simulink library "Electrical_to_Mechanical_gen"  (R2016a)
settings: Solver=ode45  StartTime=0.0  StopTime=10.0  RelTol=1e-3
undefined symbols (not defined in the file): API1dcac_efficiency, API2dcac_efficiency, API3dcac_efficiency, APIdcac_efficiency, aux_power_state, auxEmot_inertia, auxEmot_nTab_3rdD, auxEmot_power, auxEmot_pwrAC, auxEmot_Tau, auxEmot_trqTab_2ndD, auxEmot_vltTab_1stD, AWR_InvStError, DiscIntNeverNeededParam, drvEmot_emot_Cth_rotor, drvEmot_emot_Cth_stator, drvEmot_emot_dtrqEmotNeg, drvEmot_emot_dtrqEmotPtv, drvEmot_emot_inv_pwrLoss, drvEmot_emot_mot_pwrLoss, drvEmot_emot_Rth_rotor_oil, drvEmot_emot_Rth_stator_oil, drvEmot_emot_Rth_stator_rotor, drvEmot_emot_Trotor_init, drvEmot_emot_trqMaxRow, drvEmot_emot_trqMinRow, drvEmot_emot_Tstator_init, drvEmot_inv_Cth_cooling_plate, drvEmot_inv_Cth_diode, drvEmot_inv_Cth_IGBT, drvEmot_inv_n_IGBT_per_Switch, drvEmot_inv_Rth_cooling_plate_coolant, drvEmot_inv_Rth_PS_cooling_plate, drvEmot_inv_Tplate_init, drvEmot_inv_Tpowerstack_init, drvEmot_RefTqeMOT, emot_AcCmprFront_inertia, emot_AcCmprFront_nTab_3rdD, emot_AcCmprFront_pwrAC, emot_AcCmprFront_Tau, emot_AcCmprFront_trqTab_2ndD, emot_AcCmprFront_vltTab_1stD, emot_AcCmprRear_inertia, emot_AcCmprRear_nTab_3rdD, emot_AcCmprRear_pwrAC, emot_AcCmprRear_Tau, emot_AcCmprRear_trqTab_2ndD, emot_AcCmprRear_vltTab_1stD, emot_AirCmpr_inertia, emot_AirCmpr_nTab_3rdD, emot_AirCmpr_pwrAC, emot_AirCmpr_Tau, emot_AirCmpr_trqTab_2ndD, emot_AirCmpr_vltTab_1stD, emot_aircomp_power, FirstDrivenAxle_FirstDrivenAxleNoOfEmot, SecondDrivenAxle_SecondDrivenAxleNoOfEmot
libraries: Electrical_to_Mechanical_gen x4, simulink x4
(part 1 of 2)
settings Model: Creator=krishs1  LastModifiedBy=krishs1
settings DataIOCC: LimitDataPoints=on
settings DebuggingCC: AllowSymbolicDim=off

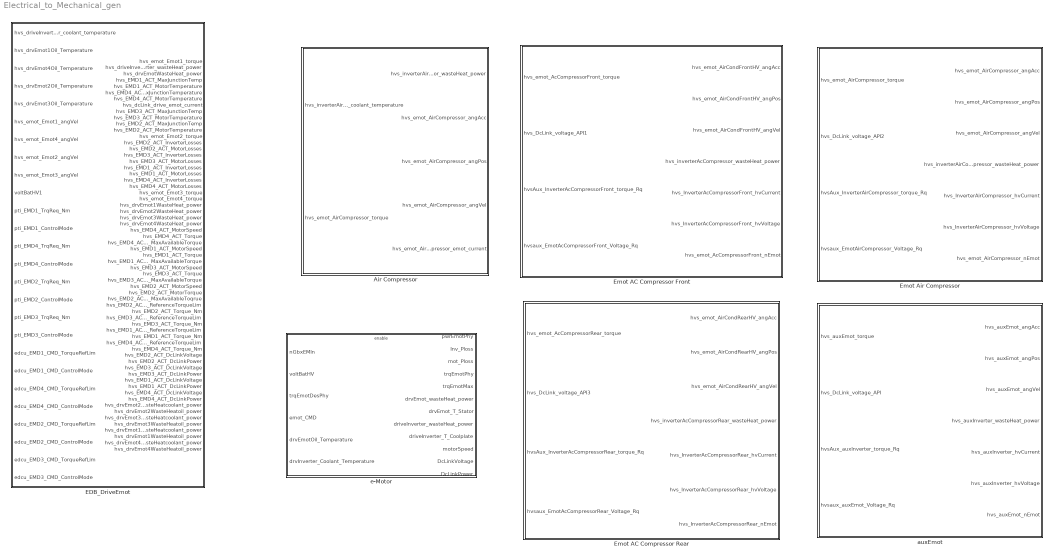
== system Electrical_to_Mechanical_gen ==
  Air Compressor : Subsystem
  EDB_DriveEmot : Subsystem
  Emot AC Compressor Front : Subsystem
  Emot AC Compressor Rear : Subsystem
  Emot Air Compressor : Subsystem
  auxEmot : Subsystem  mask{auxEmot_nTab_3rdD=auxEmot_nTab_3rdD, auxEmot_trqTab_2ndD=auxEmot_trqTab_2ndD, auxEmot_vltTab_1stD=auxEmot_vltTab_1stD, auxEmot_pwrAC=auxEmot_pwrAC, APIefficiency=1/APIdcac_efficiency, auxEmot_inertia=auxEmot_inertia, auxEmot_Tau=auxEmot_Tau, AWR_InvStError=AWR_InvStError, auxEmot_power=auxEmot_power, aux_power_state=aux_power_state}
      mask prompts: auxEmot_nTab_3rdD "Motor speed"; auxEmot_trqTab_2ndD "Motor torque"; auxEmot_vltTab_1stD "Motor voltage"; auxEmot_pwrAC "Motor power map"; APIefficiency "API efficiency"; auxEmot_inertia "Motor inertia"; AWR_InvStError "Inverter state error"; auxEmot_power "Motor average power"; aux_power_state "Switch real or constant load"
      mask TypeOptions auxEmot_nTab_3rdD: motor mode/BreakpointsForDimension1
      mask TypeOptions auxEmot_trqTab_2ndD: motor mode/BreakpointsForDimension2
      mask TypeOptions auxEmot_vltTab_1stD: motor mode/BreakpointsForDimension3
      mask TypeOptions auxEmot_pwrAC: motor mode/Table
      mask TypeOptions APIefficiency: efficiency/Gain
      mask TypeOptions auxEmot_inertia: auxEmot_inertia/Value
      mask TypeOptions AWR_InvStError: AWR_InvStError/const
      mask TypeOptions auxEmot_power: lvs_Aircomp_power/Value
      mask TypeOptions aux_power_state: switch_Real_or_Constant_Load/Value
  e-Motor : Subsystem  mask(MapModule){}

== system Electrical_to_Mechanical_gen/Air Compressor ==
  hvs_inverterAirCompressor_coolant_temperature : Inport
  hvs_emot_AirCompressor_torque : Inport  Port=2
  Constant{,1..4} (5 alike) : Constant  Value=0
  Terminator : Terminator
  Terminator1 : Terminator
  "hvs_inverterAirCompressor_wasteHeat_power " : Outport
  hvs_emot_AirCompressor_angAcc : Outport  Port=2
  hvs_emot_AirCompressor_angPos : Outport  Port=3
  hvs_emot_AirCompressor_angVel : Outport  Port=4
  hvs_emot_AirCompressor_emot_current : Outport  Port=5
  wires:
  Constant/1 -> "hvs_inverterAirCompressor_wasteHeat_power "/1
  Constant1/1 -> hvs_emot_AirCompressor_angAcc/1
  Constant2/1 -> hvs_emot_AirCompressor_angPos/1
  Constant3/1 -> hvs_emot_AirCompressor_angVel/1
  Constant4/1 -> hvs_emot_AirCompressor_emot_current/1
  hvs_inverterAirCompressor_coolant_temperature/1 -> Terminator/1
  hvs_emot_AirCompressor_torque/1 -> Terminator1/1

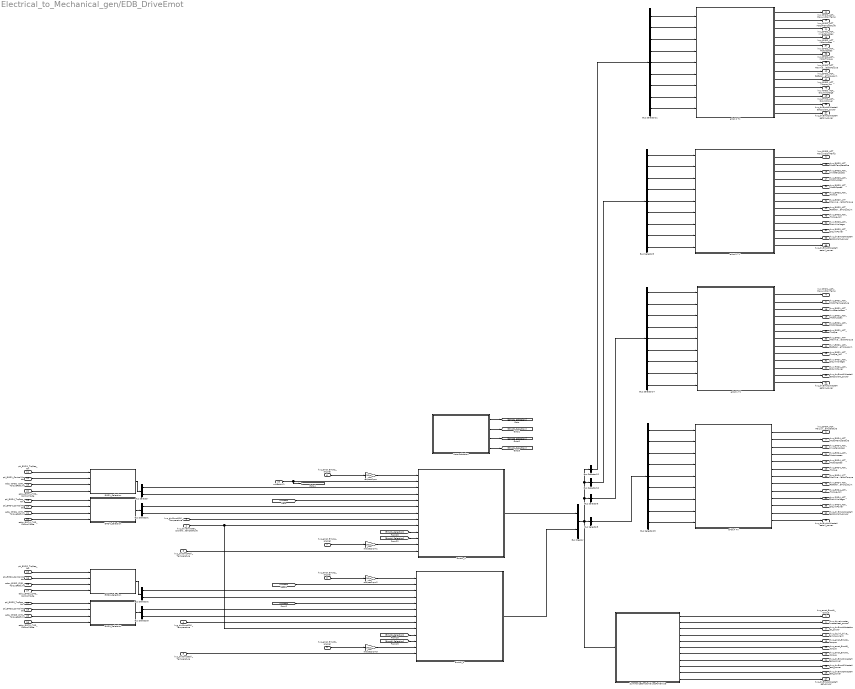
== system Electrical_to_Mechanical_gen/EDB_DriveEmot ==
  hvs_driveInverter_coolant_temperature : Inport
  hvs_drvEmot1Oil_Temperature : Inport  Port=2
  hvs_drvEmot4Oil_Temperature : Inport  Port=3
  hvs_drvEmot2Oil_Temperature : Inport  Port=4
  hvs_drvEmot3Oil_Temperature : Inport  Port=5
  hvs_emot_Emot1_angVel : Inport  Port=6
  hvs_emot_Emot4_angVel : Inport  Port=7
  hvs_emot_Emot2_angVel : Inport  Port=8
  hvs_emot_Emot3_angVel : Inport  Port=9
  voltBatHV1 : Inport  Port=10
  pti_EMD1_TrqReq_Nm : Inport  Port=11
  pti_EMD1_ControlMode : Inport  Port=12
  pti_EMD4_TrqReq_Nm : Inport  Port=13
  pti_EMD4_ControlMode : Inport  Port=14
  pti_EMD2_TrqReq_Nm : Inport  Port=15
  pti_EMD2_ControlMode : Inport  Port=16
  pti_EMD3_TrqReq_Nm : Inport  Port=17
  pti_EMD3_ControlMode : Inport  Port=18
  edcu_EMD1_CMD_TorqueRefLim : Inport  Port=19
  edcu_EMD1_CMD_ControlMode : Inport  Port=20
  edcu_EMD4_CMD_TorqueRefLim : Inport  Port=21
  edcu_EMD4_CMD_ControlMode : Inport  Port=22
  edcu_EMD2_CMD_TorqueRefLim : Inport  Port=23
  edcu_EMD2_CMD_ControlMode : Inport  Port=24
  edcu_EMD3_CMD_TorqueRefLim : Inport  Port=25
  edcu_EMD3_CMD_ControlMode : Inport  Port=26
  Bus Selector : BusSelector  OutputSignals=EMD1_TrqReq_Nm,EMD1_ControlMode
  Bus Selector1 : BusSelector  OutputSignals=EMD4_TrqReq_Nm,EMD4_ControlMode
  Bus Selector{9,11,14..15} (4 alike) : BusSelector  OutputSignals=driveInverter_T_plate,drvEmot_T_Stator,Inv_Ploss,mot_Ploss,motorSpeed,trqEmotPhy,trqEmotMax,DcLinkVoltage,DcLinkPower
  Bus Selector2 : BusSelector  OutputSignals=EMD2_TrqReq_Nm,EMD2_ControlMode
  Bus Selector3 : BusSelector  OutputSignals=EMD2_TrqReq_Nm,EMD2_ControlMode
  Bus Creator : BusCreator  Inputs=2
  Bus Selector10 : BusSelector  OutputSignals=emot2_3B.emot3B.driveInverter_T_plate,emot2_3B.emot3B.drvEmot_T_Stator,emot2_3B.emot3B.Inv_Ploss,emot2_3B.emot3B.mot_Ploss,emot2_3B.emot3B.motorSpeed,emot2_3B.emot3B.trqEmotPhy,emot2_3B.emot3B.trqEmotMax,emot2_3B.emot3B.DcLinkVoltage,emot2_3B.emot3B.DcLinkPower  OutputAsBus=on
  Bus Selector12 : BusSelector  OutputSignals=emot2_3B.emot2B.driveInverter_T_plate,emot2_3B.emot2B.drvEmot_T_Stator,emot2_3B.emot2B.Inv_Ploss,emot2_3B.emot2B.mot_Ploss,emot2_3B.emot2B.motorSpeed,emot2_3B.emot2B.trqEmotPhy,emot2_3B.emot2B.trqEmotMax,emot2_3B.emot2B.DcLinkVoltage,emot2_3B.emot2B.DcLinkPower  OutputAsBus=on
  Bus Selector5 : BusSelector  OutputSignals=emot1_4B.emot4B.motorSpeed,emot1_4B.emot4B.trqEmotPhy,emot1_4B.emot4B.trqEmotMax,emot1_4B.emot4B.driveInverter_T_plate,emot1_4B.emot4B.drvEmot_T_Stator,emot1_4B.emot4B.Inv_Ploss,emot1_4B.emot4B.mot_Ploss,emot1_4B.emot4B.DcLinkVoltage,emot1_4B.emot4B.DcLinkPower  OutputAsBus=on
  Bus Selector6 : BusSelector  OutputSignals=emot1_4B.emot1B.driveInverter_T_plate,emot1_4B.emot1B.drvEmot_T_Stator,emot1_4B.emot1B.Inv_Ploss,emot1_4B.emot1B.mot_Ploss,emot1_4B.emot1B.motorSpeed,emot1_4B.emot1B.trqEmotPhy,emot1_4B.emot1B.trqEmotMax,emot1_4B.emot1B.DcLinkVoltage,emot1_4B.emot1B.DcLinkPower  OutputAsBus=on
  EMD1_Selection : Subsystem
  EMD2_Selection : Subsystem
  EMD3_Selection : Subsystem
  EMD4_Selection : Subsystem
  Emot1_4 : Subsystem
  Emot2_3 : Subsystem
  MotorSelection : Subsystem
  SummarizeEmotorValuesForVehicle : Subsystem  TreatAsAtomicUnit=on
  eMot 1 TX : Subsystem
  eMot 2 TX : Subsystem
  eMot 3 TX : Subsystem
  eMot 4 TX : Subsystem
  rad/sec2rpm{,1..3} (4 alike) : Gain  Gain=30/pi
  hvs_emot_Emot1_torque : Outport
  hvs_driveInverter_wasteHeat_power : Outport  Port=2
  hvs_drvEmotWasteHeat_power : Outport  Port=3
  hvs_EMD1_ACT_MaxJunctionTemp : Outport  Port=4
  hvs_EMD1_ACT_MotorTemperature : Outport  Port=5
  hvs_EMD4_ACT_MaxJunctionTemperature : Outport  Port=6
  hvs_EMD4_ACT_MotorTemperature : Outport  Port=7
  hvs_dcLink_drive_emot_current : Outport  Port=8
  hvs_EMD3_ACT_MaxJunctionTemp : Outport  Port=9
  hvs_EMD3_ACT_MotorTemperature : Outport  Port=10
  hvs_EMD2_ACT_MaxJunctionTemp : Outport  Port=11
  hvs_EMD2_ACT_MotorTemperature : Outport  Port=12
  hvs_emot_Emot2_torque : Outport  Port=13
  hvs_EMD2_ACT_InverterLosses : Outport  Port=14
  hvs_EMD2_ACT_MotorLosses : Outport  Port=15
  hvs_EMD3_ACT_InverterLosses : Outport  Port=16
  hvs_EMD3_ACT_MotorLosses : Outport  Port=17
  hvs_EMD1_ACT_InverterLosses : Outport  Port=18
  hvs_EMD1_ACT_MotorLosses : Outport  Port=19
  hvs_EMD4_ACT_InverterLosses : Outport  Port=20
  hvs_EMD4_ACT_MotorLosses : Outport  Port=21
  hvs_emot_Emot3_torque : Outport  Port=22
  hvs_emot_Emot4_torque : Outport  Port=23
  hvs_drvEmot1WasteHeat_power : Outport  Port=24
  hvs_drvEmot2WasteHeat_power : Outport  Port=25
  hvs_drvEmot3WasteHeat_power : Outport  Port=26
  hvs_drvEmot4WasteHeat_power : Outport  Port=27
  hvs_EMD4_ACT_MotorSpeed : Outport  Port=28
  hvs_EMD4_ACT_Torque : Outport  Port=29
  hvs_EMD4_ACT_MaxAvailableTorque : Outport  Port=30
  hvs_EMD1_ACT_MotorSpeed : Outport  Port=31
  hvs_EMD1_ACT_Torque : Outport  Port=32
  hvs_EMD1_ACT_MaxAvailableTorque : Outport  Port=33
  hvs_EMD3_ACT_MotorSpeed : Outport  Port=34
  hvs_EMD3_ACT_Torque : Outport  Port=35
  hvs_EMD3_ACT_MaxAvailableTorque : Outport  Port=36
  hvs_EMD2_ACT_MotorSpeed : Outport  Port=37
  hvs_EMD2_ACT_MotorTorque : Outport  Port=38
  hvs_EMD2_ACT_MaxAvailableToqrue : Outport  Port=39
  hvs_EMD2_ACT_ReferenceTorqueLim : Outport  Port=40
  hvs_EMD2_ACT_Torque_Nm : Outport  Port=41
  hvs_EMD3_ACT_ReferenceTorqueLim : Outport  Port=42
  hvs_EMD3_ACT_Torque_Nm : Outport  Port=43
  hvs_EMD1_ACT_ReferenceTorqueLim : Outport  Port=44
  hvs_EMD1_ACT_Torque_Nm : Outport  Port=45
  hvs_EMD4_ACT_ReferenceTorqueLim : Outport  Port=46
  hvs_EMD4_ACT_Torque_Nm : Outport  Port=47
  hvs_EMD2_ACT_DcLinkVoltage : Outport  Port=48
  hvs_EMD2_ACT_DcLinkPower : Outport  Port=49
  hvs_EMD3_ACT_DcLinkVoltage : Outport  Port=50
  hvs_EMD3_ACT_DcLinkPower : Outport  Port=51
  hvs_EMD1_ACT_DcLinkVoltage : Outport  Port=52
  hvs_EMD1_ACT_DcLinkPower : Outport  Port=53
  hvs_EMD4_ACT_DcLinkVoltage : Outport  Port=54
  hvs_EMD4_ACT_DcLinkPower : Outport  Port=55
  hvs_drvEmot2WasteHeatcoolant_power : Outport  Port=56
  hvs_drvEmot2WasteHeatoil_power : Outport  Port=57
  hvs_drvEmot3WasteHeatcoolant_power : Outport  Port=58
  hvs_drvEmot3WasteHeatoil_power : Outport  Port=59
  hvs_drvEmot1WasteHeatcoolant_power : Outport  Port=60
  hvs_drvEmot1WasteHeatoil_power : Outport  Port=61
  hvs_drvEmot4WasteHeatcoolant_power : Outport  Port=62
  hvs_drvEmot4WasteHeatoil_power : Outport  Port=63
  wires:
  eMot 4 TX/11(hvs_EMD4_ACT_DcLinkPower) -> hvs_EMD4_ACT_DcLinkPower/1
  eMot 4 TX/10(hvs_EMD4_ACT_DcLinkVoltage) -> hvs_EMD4_ACT_DcLinkVoltage/1
  Bus Selector15/9 -> eMot 4 TX/9(IN_EMD4_ACT_DcLinkPower)  "<DcLinkPower>"
  Bus Selector15/8 -> eMot 4 TX/8(IN_EMD4_ACT_DcLinkVoltage)  "<DcLinkVoltage>"
  eMot 1 TX/11(hvs_EMD1_ACT_DcLinkPower) -> hvs_EMD1_ACT_DcLinkPower/1
  eMot 1 TX/10(hvs_EMD1_ACT_DcLinkVoltage) -> hvs_EMD1_ACT_DcLinkVoltage/1
  Bus Selector14/9 -> eMot 1 TX/9(IN_EMD1_ACT_DcLinkPower)  "<DcLinkPower>"
  Bus Selector14/8 -> eMot 1 TX/8(IN_EMD1_ACT_DcLinkVoltage)  "<DcLinkVoltage>"
  eMot 3 TX/11(hvs_EMD3_ACT_DcLinkPower) -> hvs_EMD3_ACT_DcLinkPower/1
  eMot 3 TX/10(hvs_EMD3_ACT_DcLinkVoltage) -> hvs_EMD3_ACT_DcLinkVoltage/1
  Bus Selector9/8 -> eMot 3 TX/8(IN_EMD3_ACT_DcLinkVoltage)  "<DcLinkVoltage>"
  Bus Selector9/9 -> eMot 3 TX/9(IN_EMD3_ACT_DcLinkPower)  "<DcLinkPower>"
  eMot 2 TX/11(hvs_EMD2_ACT_DcLinkPower) -> hvs_EMD2_ACT_DcLinkPower/1
  eMot 2 TX/10(hvs_EMD2_ACT_DcLinkVoltage) -> hvs_EMD2_ACT_DcLinkVoltage/1
  Bus Selector11/9 -> eMot 2 TX/9(IN_EMD2_ACT_DcLinkPower)  "<DcLinkPower>"
  Bus Selector11/8 -> eMot 2 TX/8(IN_EMD2_ACT_DcLinkVoltage)  "<DcLinkVoltage>"
  Bus Selector2/2 -> Emot2_3/4(emot_CMD2)  "<EMD2_ControlMode>"
  Bus Selector2/1 -> Emot2_3/3(trqEmotDesPhy2)  "<EMD2_TrqReq_Nm>"
  Bus Selector3/1 -> Emot2_3/6(trqEmotDesPhy3)  "<EMD2_TrqReq_Nm>"
  Bus Selector3/2 -> Emot2_3/7(emot_CMD3)  "<EMD2_ControlMode>"
  pti_EMD3_ControlMode/1 -> EMD3_Selection/2(pti_EMD2_ControlMode)
  pti_EMD3_TrqReq_Nm/1 -> EMD3_Selection/1(pti_EMD2_TrqReq_Nm)
  EMD3_Selection/1(Signal) -> Bus Selector3/1
  edcu_EMD3_CMD_ControlMode/1 -> EMD3_Selection/4(edcu_EMD2_CMD_ControlMode)
  edcu_EMD3_CMD_TorqueRefLim/1 -> EMD3_Selection/3(edcu_EMD2_CMD_TorqueRefLim)
  EMD2_Selection/1(Signal) -> Bus Selector2/1
  edcu_EMD2_CMD_ControlMode/1 -> EMD2_Selection/4(edcu_EMD2_CMD_ControlMode)
  edcu_EMD2_CMD_TorqueRefLim/1 -> EMD2_Selection/3(edcu_EMD2_CMD_TorqueRefLim)
  pti_EMD2_ControlMode/1 -> EMD2_Selection/2(pti_EMD2_ControlMode)
  pti_EMD2_TrqReq_Nm/1 -> EMD2_Selection/1(pti_EMD2_TrqReq_Nm)
  Bus Selector1/2 -> Emot1_4/7(emot_CMD4)  "<EMD4_ControlMode>"
  Bus Selector1/1 -> Emot1_4/6(trqEmotDesPhy4)  "<EMD4_TrqReq_Nm>"
  EMD4_Selection/1(Signal) -> Bus Selector1/1
  edcu_EMD4_CMD_ControlMode/1 -> EMD4_Selection/4(edcu_EMD4_CMD_ControlMode)
  edcu_EMD4_CMD_TorqueRefLim/1 -> EMD4_Selection/3(edcu_EMD4_CMD_TorqueRefLim)
  Bus Selector/2 -> Emot1_4/4(emot_CMD1)  "<EMD1_ControlMode>"
  Bus Selector/1 -> Emot1_4/3(trqEmotDesPhy1)  "<EMD1_TrqReq_Nm>"
  EMD1_Selection/1(Signal) -> Bus Selector/1
  edcu_EMD1_CMD_ControlMode/1 -> EMD1_Selection/4(edcu_EMD1_CMD_ControlMode)
  edcu_EMD1_CMD_TorqueRefLim/1 -> EMD1_Selection/3(edcu_EMD1_CMD_TorqueRefLim)
  pti_EMD1_ControlMode/1 -> EMD1_Selection/2(pti_EMD1_ControlMode)
  pti_EMD1_TrqReq_Nm/1 -> EMD1_Selection/1(pti_EMD1_TrqReq_Nm)
  eMot 4 TX/9(hvs_EMD4_ACT_Torque_Nm) -> hvs_EMD4_ACT_Torque_Nm/1
  eMot 4 TX/8(hvs_EMD4_ACT_ReferenceTorqueLim) -> hvs_EMD4_ACT_ReferenceTorqueLim/1
  eMot 1 TX/9(hvs_EMD1_ACT_Torque_Nm) -> hvs_EMD1_ACT_Torque_Nm/1
  eMot 1 TX/8(hvs_EMD1_ACT_ReferenceTorqueLim) -> hvs_EMD1_ACT_ReferenceTorqueLim/1
  eMot 3 TX/9(hvs_EMD3_ACT_Torque_Nm) -> hvs_EMD3_ACT_Torque_Nm/1
  eMot 3 TX/8(hvs_EMD3_ACT_ReferenceTorqueLim) -> hvs_EMD3_ACT_ReferenceTorqueLim/1
  eMot 2 TX/8(hvs_EMD2_ACT_ReferenceTorqueLim) -> hvs_EMD2_ACT_ReferenceTorqueLim/1
  eMot 2 TX/9(hvs_EMD2_ACT_Torque_Nm) -> hvs_EMD2_ACT_Torque_Nm/1
  rad/sec2rpm3/1 -> Emot2_3/12(hvs_emot_Emot3_angVel)
  rad/sec2rpm2/1 -> Emot2_3/1(hvs_emot_Emot2_angVel)
  rad/sec2rpm1/1 -> Emot1_4/12(hvs_emot_Emot4_angVel)
  rad/sec2rpm/1 -> Emot1_4/1(hvs_emot_Emot1_angVel)
  [voltBat] -> Emot2_3/5(voltBatHV3)
  [voltBat] -> Emot2_3/2(voltBatHV2)
  pti_EMD4_ControlMode/1 -> EMD4_Selection/2(pti_EMD4_ControlMode)
  pti_EMD4_TrqReq_Nm/1 -> EMD4_Selection/1(pti_EMD4_TrqReq_Nm)
  [voltBat] -> Emot1_4/5(voltBatHV4)
  voltBatHV1/1 -> [voltBat], Emot1_4/2(voltBatHV1)
  hvs_emot_Emot3_angVel/1 -> rad/sec2rpm3/1
  hvs_emot_Emot2_angVel/1 -> rad/sec2rpm2/1
  hvs_emot_Emot4_angVel/1 -> rad/sec2rpm1/1
  hvs_emot_Emot1_angVel/1 -> rad/sec2rpm/1
  SummarizeEmotorValuesForVehicle/11(hvs_drvEmot4WasteHeat_power) -> hvs_drvEmot4WasteHeat_power/1
  SummarizeEmotorValuesForVehicle/10(hvs_drvEmot3WasteHeat_power) -> hvs_drvEmot3WasteHeat_power/1
  SummarizeEmotorValuesForVehicle/9(hvs_drvEmot2WasteHeat_power) -> hvs_drvEmot2WasteHeat_power/1
  SummarizeEmotorValuesForVehicle/8(hvs_drvEmot1WasteHeat_power) -> hvs_drvEmot1WasteHeat_power/1
  hvs_drvEmot3Oil_Temperature/1 -> Emot2_3/13(hvs_drvEmot3Oil_Temperature)
  hvs_drvEmot2Oil_Temperature/1 -> Emot2_3/8(hvs_drvEmot2Oil_Temperature)
  hvs_drvEmot4Oil_Temperature/1 -> Emot1_4/13(hvs_drvEmot4Oil_Temperature)
  SummarizeEmotorValuesForVehicle/7(hvs_emot_Emot4_torque) -> hvs_emot_Emot4_torque/1
  SummarizeEmotorValuesForVehicle/6(hvs_emot_Emot3_torque) -> hvs_emot_Emot3_torque/1
  [Emot3_Selection] -> Emot2_3/11(Emot3_Selection)
  [Emot2_Selection] -> Emot2_3/10(Emot2_Selection)
  [Emot4_Selection] -> Emot1_4/11(Emot4_Selection)
  [Emot1_Selection] -> Emot1_4/10(Emot1_Selection)
  MotorSelection/4(Emot4_Selection) -> [Emot4_Selection]
  MotorSelection/3(Emot3_Selection) -> [Emot3_Selection]
  MotorSelection/2(Emot2_Selection) -> [Emot2_Selection]
  MotorSelection/1(Emot1_Selection) -> [Emot1_Selection]
  Bus Selector15/4 -> eMot 4 TX/4(IN_EMD4_ACT_MotorLosses)  "<mot_Ploss>"
  Bus Selector15/3 -> eMot 4 TX/3(IN_EMD4_ACT_InverterLosses)  "<Inv_Ploss>"
  eMot 4 TX/4(hvs_EMD4_ACT_MotorLosses) -> hvs_EMD4_ACT_MotorLosses/1
  eMot 4 TX/3(hvs_EMD4_ACT_InverterLosses) -> hvs_EMD4_ACT_InverterLosses/1
  Bus Selector9/4 -> eMot 3 TX/4(IN_EMD3_ACT_MotorLosses)  "<mot_Ploss>"
  Bus Selector9/3 -> eMot 3 TX/3(IN_EMD3_ACT_InverterLosses)  "<Inv_Ploss>"
  eMot 3 TX/4(hvs_EMD3_ACT_MotorLosses) -> hvs_EMD3_ACT_MotorLosses/1
  eMot 3 TX/3(hvs_EMD3_ACT_InverterLosses) -> hvs_EMD3_ACT_InverterLosses/1
  eMot 2 TX/4(hvs_EMD2_ACT_MotorLosses) -> hvs_EMD2_ACT_MotorLosses/1
  eMot 2 TX/3(hvs_EMD2_ACT_InverterLosses) -> hvs_EMD2_ACT_InverterLosses/1
  eMot 1 TX/4(hvs_EMD1_ACT_MotorLosses) -> hvs_EMD1_ACT_MotorLosses/1
  eMot 1 TX/3(hvs_EMD1_ACT_InverterLosses) -> hvs_EMD1_ACT_InverterLosses/1
  Bus Selector14/4 -> eMot 1 TX/4(IN_EMD1_ACT_MotorLosses)  "<mot_Ploss>"
  Bus Selector14/3 -> eMot 1 TX/3(IN_EMD1_ACT_InverterLosses)  "<Inv_Ploss>"
  Bus Selector11/4 -> eMot 2 TX/4(IN_EMD2_ACT_MotorLosses)  "<mot_Ploss>"
  Bus Selector11/3 -> eMot 2 TX/3(IN_EMD2_ACT_InverterLosses)  "<Inv_Ploss>"
  SummarizeEmotorValuesForVehicle/5(hvs_emot_Emot2_torque) -> hvs_emot_Emot2_torque/1
  eMot 2 TX/2(hvs_EMD2_ACT_MotorTemperature) -> hvs_EMD2_ACT_MotorTemperature/1
  eMot 2 TX/1(hvs_EMD2_ACT_MaxJunctionTemp) -> hvs_EMD2_ACT_MaxJunctionTemp/1
  Bus Selector12/1 -> Bus Selector11/1  "TransInt"
  Bus Selector11/1 -> eMot 2 TX/1(IN_EMD2_ACT_MaxJunctionTemperature)  "<driveInverter_T_plate>"
  Bus Selector11/2 -> eMot 2 TX/2(IN_EMD2_ACT_MotorTemperature)  "<drvEmot_T_Stator>"
  eMot 3 TX/2(hvs_EMD3_ACT_MotorTemperature) -> hvs_EMD3_ACT_MotorTemperature/1
  eMot 3 TX/1(hvs_EMD3_ACT_MaxJunctionTemp) -> hvs_EMD3_ACT_MaxJunctionTemp/1
  Bus Selector10/1 -> Bus Selector9/1  "TransInt"
  Bus Selector9/1 -> eMot 3 TX/1(IN_EMD3_ACT_MaxJunctionTemperature)  "<driveInverter_T_plate>"
  Bus Selector9/2 -> eMot 3 TX/2(IN_EMD3_ACT_MotorTemperature)  "<drvEmot_T_Stator>"
  Emot2_3/1(emot2_3B) -> Bus Creator/2
  Emot1_4/1(emot1_4B) -> Bus Creator/1
  SummarizeEmotorValuesForVehicle/2(hvs_driveInverter_wasteHeat_power) -> hvs_driveInverter_wasteHeat_power/1
  SummarizeEmotorValuesForVehicle/3(hvs_drvEmotWasteHeat_power) -> hvs_drvEmotWasteHeat_power/1
  eMot 4 TX/2(hvs_EMD4_ACT_MotorTemperature) -> hvs_EMD4_ACT_MotorTemperature/1
  eMot 4 TX/1(hvs_EMD4_ACT_MaxJunctionTemperature) -> hvs_EMD4_ACT_MaxJunctionTemperature/1
  eMot 1 TX/2(hvs_EMD1_ACT_MotorTemperature) -> hvs_EMD1_ACT_MotorTemperature/1
  eMot 1 TX/1(hvs_EMD1_ACT_MaxJunctionTemp) -> hvs_EMD1_ACT_MaxJunctionTemp/1
  SummarizeEmotorValuesForVehicle/4(hvs_dcLink_drive_emot_current) -> hvs_dcLink_drive_emot_current/1
  SummarizeEmotorValuesForVehicle/1(hvs_emot_Emot1_torque) -> hvs_emot_Emot1_torque/1
  Bus Selector6/1 -> Bus Selector14/1  "TransInt"
  Bus Selector15/1 -> eMot 4 TX/1(IN_EMD4_ACT_MaxJunctionTemperature)  "<driveInverter_T_plate>"
  Bus Selector15/2 -> eMot 4 TX/2(IN_EMD4_ACT_MotorTemperature)  "<drvEmot_T_Stator>"
  Bus Creator/1 -> Bus Selector6/1, Bus Selector10/1, Bus Selector12/1, Bus Selector5/1, SummarizeEmotorValuesForVehicle/1(MultiBus_Emot_Inv_1_4)
  Bus Selector14/1 -> eMot 1 TX/1(IN_EMD1_ACT_MaxJunctionTemperature)  "<driveInverter_T_plate>"
  Bus Selector14/2 -> eMot 1 TX/2(IN_EMD1_ACT_MotorTemperature)  "<drvEmot_T_Stator>"
  Bus Selector5/1 -> Bus Selector15/1  "TransInt"
  hvs_drvEmot1Oil_Temperature/1 -> Emot1_4/8(hvs_drvEmot1Oil_Temperature)
  hvs_driveInverter_coolant_temperature/1 -> Emot1_4/9(inv_coolant_temperature), Emot2_3/9(inv_coolant_temperature)
  Bus Selector15/5 -> eMot 4 TX/5(IN_EMD4_ACT_MotorSpeed)  "<motorSpeed>"
  Bus Selector15/6 -> eMot 4 TX/6(IN_EMD4_ACT_Torque)  "<trqEmotPhy>"
  Bus Selector15/7 -> eMot 4 TX/7(IN_EMD4_ACT_MaximumAvailableTorque)  "<trqEmotMax>"
  eMot 4 TX/5(hvs_EMD4_ACT_MotorSpeed) -> hvs_EMD4_ACT_MotorSpeed/1
  eMot 4 TX/6(hvs_EMD4_ACT_Torque) -> hvs_EMD4_ACT_Torque/1
  eMot 4 TX/7(hvs_EMD4_ACT_MaxAvailableTorque) -> hvs_EMD4_ACT_MaxAvailableTorque/1
  Bus Selector14/5 -> eMot 1 TX/5(IN_EMD1_ACT_MotorSpeed)  "<motorSpeed>"
  Bus Selector14/6 -> eMot 1 TX/6(IN_EMD1_ACT_Torque)  "<trqEmotPhy>"
  Bus Selector14/7 -> eMot 1 TX/7(IN_EMD1_ACT_MaximumAvailableTorque)  "<trqEmotMax>"
  eMot 1 TX/5(hvs_EMD1_ACT_MotorSpeed) -> hvs_EMD1_ACT_MotorSpeed/1
  eMot 1 TX/6(hvs_EMD1_ACT_Torque) -> hvs_EMD1_ACT_Torque/1
  eMot 1 TX/7(hvs_EMD1_ACT_MaxAvailableTorque) -> hvs_EMD1_ACT_MaxAvailableTorque/1
  Bus Selector9/5 -> eMot 3 TX/5(IN_EMD3_ACT_MotorSpeed)  "<motorSpeed>"
  Bus Selector9/6 -> eMot 3 TX/6(IN_EMD3_ACT_Torque)  "<trqEmotPhy>"
  Bus Selector9/7 -> eMot 3 TX/7(IN_EMD3_ACT_MaximumAvailableTorque)  "<trqEmotMax>"
  eMot 3 TX/5(hvs_EMD3_ACT_MotorSpeed) -> hvs_EMD3_ACT_MotorSpeed/1
  eMot 3 TX/6(hvs_EMD3_ACT_Torque) -> hvs_EMD3_ACT_Torque/1
  eMot 3 TX/7(hvs_EMD3_ACT_MaxAvailableTorque) -> hvs_EMD3_ACT_MaxAvailableTorque/1
  Bus Selector11/5 -> eMot 2 TX/5(IN_EMD2_ACT_MotorSpeed)  "<motorSpeed>"
  Bus Selector11/6 -> eMot 2 TX/6(IN_EMD2_ACT_Torque)  "<trqEmotPhy>"
  Bus Selector11/7 -> eMot 2 TX/7(IN_EMD2_ACT_MaximumAvailableTorque)  "<trqEmotMax>"
  eMot 2 TX/5(hvs_EMD2_ACT_MotorSpeed) -> hvs_EMD2_ACT_MotorSpeed/1
  eMot 2 TX/6(hvs_EMD2_ACT_Torque) -> hvs_EMD2_ACT_MotorTorque/1
  eMot 2 TX/7(hvs_EMD2_ACT_MaxAvailableTorque) -> hvs_EMD2_ACT_MaxAvailableToqrue/1
  eMot 2 TX/12(hvs_drvEmot2WasteHeatcoolant_power) -> hvs_drvEmot2WasteHeatcoolant_power/1
  eMot 2 TX/13(hvs_drvEmot2WasteHeatoil_power) -> hvs_drvEmot2WasteHeatoil_power/1
  eMot 3 TX/12(hvs_drvEmot3WasteHeatcoolant_power) -> hvs_drvEmot3WasteHeatcoolant_power/1
  eMot 3 TX/13(hvs_drvEmot3WasteHeatoil_power) -> hvs_drvEmot3WasteHeatoil_power/1
  eMot 1 TX/12(hvs_drvEmot1WasteHeatcoolant_power) -> hvs_drvEmot1WasteHeatcoolant_power/1
  eMot 1 TX/13(hvs_drvEmot1WasteHeatoil_power) -> hvs_drvEmot1WasteHeatoil_power/1
  eMot 4 TX/13(hvs_drvEmot4WasteHeatoil_power) -> hvs_drvEmot4WasteHeatoil_power/1
  eMot 4 TX/12(hvs_drvEmot4WasteHeatcoolant_power) -> hvs_drvEmot4WasteHeatcoolant_power/1

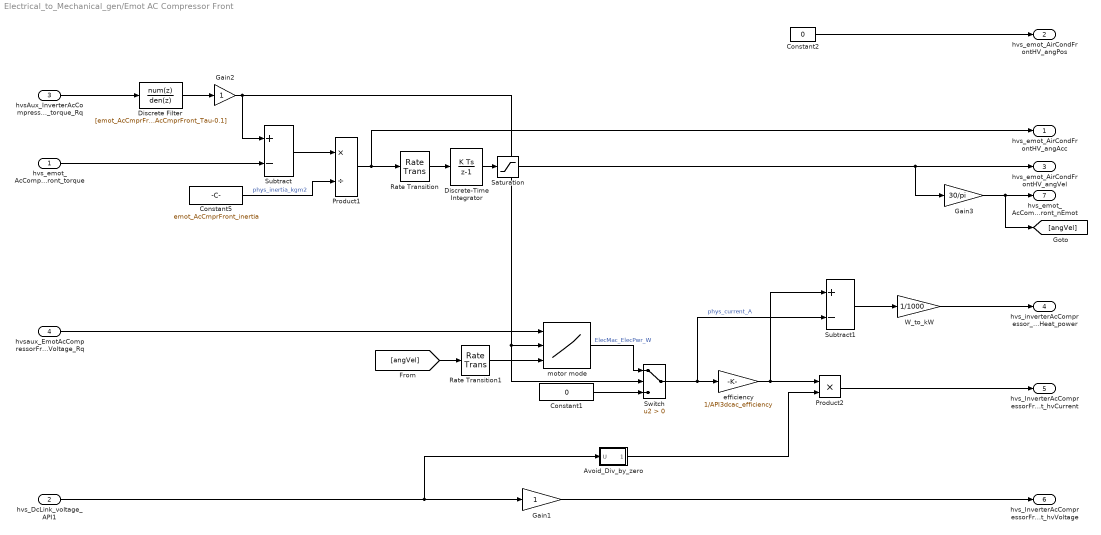
== system Electrical_to_Mechanical_gen/Emot AC Compressor Front ==
  hvs_emot_AcCompressorFront_torque : Inport
  hvs_DcLink_voltage_API1 : Inport  Port=2
  hvsAux_InverterAcCompressorFront_torque_Rq : Inport  Port=3
  hvsaux_EmotAcCompressorFront_Voltage_Rq : Inport  Port=4
  Avoid_Div_by_zero : Subsystem
  Constant1 : Constant  Value=0
  Constant2 : Constant  Value=0
  Constant5 : Constant  Value=emot_AcCmprFront_inertia
  Discrete Filter : DiscreteFilter  Numerator=[emot_AcCmprFront_Tau emot_AcCmprFront_Tau]  Denominator=[0.1+emot_AcCmprFront_Tau emot_AcCmprFront_Tau-0.1]
  Discrete-Time Integrator : DiscreteIntegrator  SampleTime=-1  ICPrevOutput=DiscIntNeverNeededParam  ICPrevScaledInput=DiscIntNeverNeededParam
  Gain1 : Gain
      settings: AttributesFormatString=%<Description>
  Gain2 : Gain
      mask init:
      | K = str2num(get_param(bdroot,'FixedStep'));
  Gain3 : Gain  Gain=30/pi
      settings: AttributesFormatString=%<Description>
  Product1 : Product  Inputs=*/  RndMeth=Zero
  Product2 : Product  Inputs=**  RndMeth=Zero
  Rate Transition : RateTransition
  Rate Transition1 : RateTransition
  Saturation : Saturate  UpperLimit=Inf  LowerLimit=0
  Subtract : Sum  Inputs=+-
  Subtract1 : Sum  Inputs=+-
  Switch : Switch  Criteria=u2 > Threshold
  W_to_kW : Gain  Gain=1/1000
      settings: AttributesFormatString=%<Description>
  efficiency : Gain  Gain=1/API3dcac_efficiency
      settings: AttributesFormatString=%<Description>
  motor mode : Lookup_n-D  NumberOfTableDimensions=3  BreakpointsForDimension1=emot_AcCmprFront_vltTab_1stD  BreakpointsForDimension2=emot_AcCmprFront_trqTab_2ndD  BreakpointsForDimension3=emot_AcCmprFront_nTab_3rdD  Table=emot_AcCmprFront_pwrAC  ExtrapMethod=Clip  UseLastTableValue=on  InputSameDT=on
  hvs_emot_AirCondFrontHV_angAcc : Outport
  hvs_emot_AirCondFrontHV_angPos : Outport  Port=2
  hvs_emot_AirCondFrontHV_angVel : Outport  Port=3
  hvs_inverterAcCompressor_wasteHeat_power : Outport  Port=4
  hvs_InverterAcCompressorFront_hvCurrent : Outport  Port=5
  hvs_InverterAcCompressorFront_hvVoltage : Outport  Port=6
  hvs_emot_AcCompressorFront_nEmot : Outport  Port=7
  wires:
  W_to_kW/1 -> hvs_inverterAcCompressor_wasteHeat_power/1
  Gain2/1 -> Switch/2, motor mode/2, Subtract/1
  Subtract1/1 -> W_to_kW/1
  efficiency/1 -> Product2/1, Subtract1/1
  Switch/1 -> efficiency/1, Subtract1/2  "phys_current_A"
  Product2/1 -> hvs_InverterAcCompressorFront_hvCurrent/1
  Avoid_Div_by_zero/1(1/U) -> Product2/2
  hvs_DcLink_voltage_API1/1 -> Gain1/1, Avoid_Div_by_zero/1(U)
  Gain1/1 -> hvs_InverterAcCompressorFront_hvVoltage/1
  Constant1/1 -> Switch/3
  Constant2/1 -> hvs_emot_AirCondFrontHV_angPos/1
  hvsAux_InverterAcCompressorFront_torque_Rq/1 -> Discrete Filter/1
  hvsaux_EmotAcCompressorFront_Voltage_Rq/1 -> motor mode/1
  motor mode/1 -> Switch/1  "ElecMac_ElecPwr_W"
  Discrete Filter/1 -> Gain2/1
  hvs_emot_AcCompressorFront_torque/1 -> Subtract/2
  Subtract/1 -> Product1/1
  Constant5/1 -> Product1/2  "phys_inertia_kgm2"
  Product1/1 -> hvs_emot_AirCondFrontHV_angAcc/1, Rate Transition/1
  Discrete-Time Integrator/1 -> Saturation/1
  Saturation/1 -> hvs_emot_AirCondFrontHV_angVel/1, Gain3/1
  Rate Transition/1 -> Discrete-Time Integrator/1
  [angVel] -> Rate Transition1/1
  Rate Transition1/1 -> motor mode/3
  Gain3/1 -> hvs_emot_AcCompressorFront_nEmot/1, [angVel]

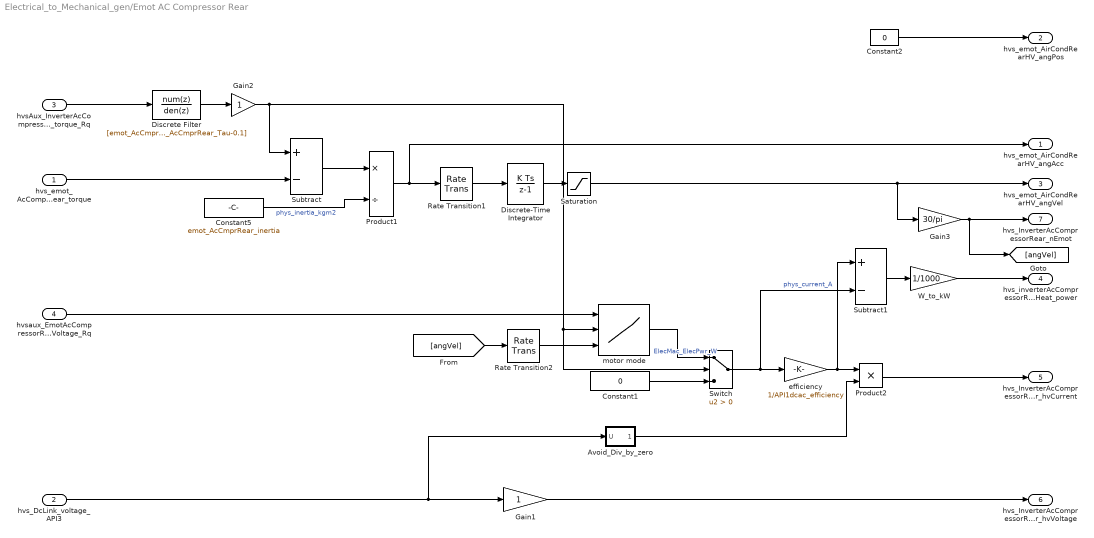
== system Electrical_to_Mechanical_gen/Emot AC Compressor Rear ==
  hvs_emot_AcCompressorRear_torque : Inport
  hvs_DcLink_voltage_API3 : Inport  Port=2
  hvsAux_InverterAcCompressorRear_torque_Rq : Inport  Port=3
  hvsaux_EmotAcCompressorRear_Voltage_Rq : Inport  Port=4
  Avoid_Div_by_zero : Subsystem
  Constant1 : Constant  Value=0
  Constant2 : Constant  Value=0
  Constant5 : Constant  Value=emot_AcCmprRear_inertia
  Discrete Filter : DiscreteFilter  Numerator=[emot_AcCmprRear_Tau emot_AcCmprRear_Tau]  Denominator=[0.1+emot_AcCmprRear_Tau emot_AcCmprRear_Tau-0.1]
  Discrete-Time Integrator : DiscreteIntegrator  SampleTime=-1  ICPrevOutput=DiscIntNeverNeededParam  ICPrevScaledInput=DiscIntNeverNeededParam
  Gain1 : Gain
      settings: AttributesFormatString=%<Description>
  Gain2 : Gain
      mask init:
      | K = str2num(get_param(bdroot,'FixedStep'));
  Gain3 : Gain  Gain=30/pi
      settings: AttributesFormatString=%<Description>
  Product1 : Product  Inputs=*/  RndMeth=Zero
  Product2 : Product  Inputs=**  RndMeth=Zero
  Rate Transition1 : RateTransition
  Rate Transition2 : RateTransition
  Saturation : Saturate  UpperLimit=Inf  LowerLimit=0
  Subtract : Sum  Inputs=+-
  Subtract1 : Sum  Inputs=+-
  Switch : Switch  Criteria=u2 > Threshold
  W_to_kW : Gain  Gain=1/1000
      settings: AttributesFormatString=%<Description>
  efficiency : Gain  Gain=1/API1dcac_efficiency
      settings: AttributesFormatString=%<Description>
  motor mode : Lookup_n-D  NumberOfTableDimensions=3  BreakpointsForDimension1=emot_AcCmprRear_vltTab_1stD  BreakpointsForDimension2=emot_AcCmprRear_trqTab_2ndD  BreakpointsForDimension3=emot_AcCmprRear_nTab_3rdD  Table=emot_AcCmprRear_pwrAC  ExtrapMethod=Clip  UseLastTableValue=on  InputSameDT=on
  hvs_emot_AirCondRearHV_angAcc : Outport
  hvs_emot_AirCondRearHV_angPos : Outport  Port=2
  hvs_emot_AirCondRearHV_angVel : Outport  Port=3
  hvs_inverterAcCompressorRear_wasteHeat_power : Outport  Port=4
  hvs_InverterAcCompressorRear_hvCurrent : Outport  Port=5
  hvs_InverterAcCompressorRear_hvVoltage : Outport  Port=6
  hvs_InverterAcCompressorRear_nEmot : Outport  Port=7
  wires:
  W_to_kW/1 -> hvs_inverterAcCompressorRear_wasteHeat_power/1
  Gain2/1 -> Subtract/1, Switch/2, motor mode/2
  Subtract1/1 -> W_to_kW/1
  efficiency/1 -> Subtract1/1, Product2/1
  Switch/1 -> efficiency/1, Subtract1/2  "phys_current_A"
  Avoid_Div_by_zero/1(1/U) -> Product2/2
  Product2/1 -> hvs_InverterAcCompressorRear_hvCurrent/1
  Gain1/1 -> hvs_InverterAcCompressorRear_hvVoltage/1
  hvs_DcLink_voltage_API3/1 -> Gain1/1, Avoid_Div_by_zero/1(U)
  Constant1/1 -> Switch/3
  Saturation/1 -> hvs_emot_AirCondRearHV_angVel/1, Gain3/1
  Discrete-Time Integrator/1 -> Saturation/1
  Product1/1 -> Rate Transition1/1, hvs_emot_AirCondRearHV_angAcc/1
  Constant5/1 -> Product1/2  "phys_inertia_kgm2"
  Subtract/1 -> Product1/1
  hvs_emot_AcCompressorRear_torque/1 -> Subtract/2
  Discrete Filter/1 -> Gain2/1
  motor mode/1 -> Switch/1  "ElecMac_ElecPwr_W"
  hvsaux_EmotAcCompressorRear_Voltage_Rq/1 -> motor mode/1
  hvsAux_InverterAcCompressorRear_torque_Rq/1 -> Discrete Filter/1
  Constant2/1 -> hvs_emot_AirCondRearHV_angPos/1
  Rate Transition1/1 -> Discrete-Time Integrator/1
  [angVel] -> Rate Transition2/1
  Rate Transition2/1 -> motor mode/3
  Gain3/1 -> [angVel], hvs_InverterAcCompressorRear_nEmot/1

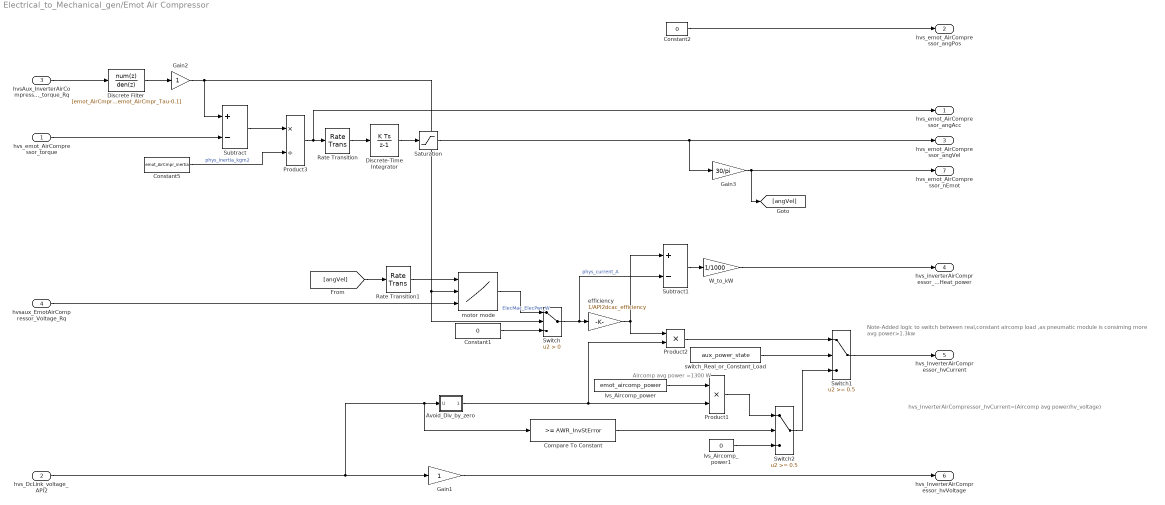
== system Electrical_to_Mechanical_gen/Emot Air Compressor ==
  note: Note-Added logic to switch between real,constant aircomp load ,as pneumatic module is consiming more avg power>1.3kw
  note: hvs_InverterAirCompressor_hvCurrent=(Aircomp avg power/hv_voltage)
  note: Aircomp avg power =1300 W
  hvs_emot_AirCompressor_torque : Inport
  hvs_DcLink_voltage_API2 : Inport  Port=2
  hvsAux_InverterAirCompressor_torque_Rq : Inport  Port=3
  hvsaux_EmotAirCompressor_Voltage_Rq : Inport  Port=4
  Avoid_Div_by_zero : Subsystem
  Compare To Constant : simulink/Logic and Bit Operations/Compare To Constant  relop=>=  const=AWR_InvStError  OutDataTypeStr=boolean
  Constant1 : Constant  Value=0
  Constant2 : Constant  Value=0
  Constant5 : Constant  Value=emot_AirCmpr_inertia
  Discrete Filter : DiscreteFilter  Numerator=[emot_AirCmpr_Tau emot_AirCmpr_Tau]  Denominator=[0.1+emot_AirCmpr_Tau emot_AirCmpr_Tau-0.1]
  Discrete-Time Integrator : DiscreteIntegrator  SampleTime=-1  ICPrevOutput=DiscIntNeverNeededParam  ICPrevScaledInput=DiscIntNeverNeededParam
  Gain1 : Gain
      settings: AttributesFormatString=%<Description>
  Gain2 : Gain
      mask init:
      | K = str2num(get_param(bdroot,'FixedStep'));
  Gain3 : Gain  Gain=30/pi
      settings: AttributesFormatString=%<Description>
  Product1 : Product  Inputs=**  RndMeth=Zero
  Product2 : Product  Inputs=**  RndMeth=Zero
  Product3 : Product  Inputs=*/  RndMeth=Zero
  Rate Transition : RateTransition
  Rate Transition1 : RateTransition
  Saturation : Saturate  UpperLimit=inf  LowerLimit=0
  Subtract : Sum  Inputs=+-
  Subtract1 : Sum  Inputs=+-
  Switch : Switch  Criteria=u2 > Threshold
  Switch1 : Switch  Threshold=0.5
  Switch2 : Switch  Threshold=0.5
  W_to_kW : Gain  Gain=1/1000
      settings: AttributesFormatString=%<Description>
  efficiency : Gain  Gain=1/API2dcac_efficiency
      settings: AttributesFormatString=%<Description>
  lvs_Aircomp_power : Constant  Value=emot_aircomp_power
  lvs_Aircomp_power1 : Constant  Value=0
  motor mode : Lookup_n-D  NumberOfTableDimensions=3  BreakpointsForDimension1=emot_AirCmpr_nTab_3rdD  BreakpointsForDimension2=emot_AirCmpr_trqTab_2ndD  BreakpointsForDimension3=emot_AirCmpr_vltTab_1stD  Table=emot_AirCmpr_pwrAC  ExtrapMethod=Clip  UseLastTableValue=on  InputSameDT=on
  switch_Real_or_Constant_Load : Constant  Value=aux_power_state
  hvs_emot_AirCompressor_angAcc : Outport
  hvs_emot_AirCompressor_angPos : Outport  Port=2
  hvs_emot_AirCompressor_angVel : Outport  Port=3
  hvs_inverterAirCompressor_wasteHeat_power : Outport  Port=4
  hvs_InverterAirCompressor_hvCurrent : Outport  Port=5
  hvs_InverterAirCompressor_hvVoltage : Outport  Port=6
  hvs_emot_AirCompressor_nEmot : Outport  Port=7
  wires:
  Switch2/1 -> Switch1/3
  Product1/1 -> Switch2/1
  Compare To Constant/1 -> Switch2/2
  lvs_Aircomp_power/1 -> Product1/1
  lvs_Aircomp_power1/1 -> Switch2/3
  hvs_DcLink_voltage_API2/1 -> Gain1/1, Avoid_Div_by_zero/1(U), Compare To Constant/1
  switch_Real_or_Constant_Load/1 -> Switch1/2
  Product2/1 -> Switch1/1
  Gain3/1 -> hvs_emot_AirCompressor_nEmot/1, [angVel]
  W_to_kW/1 -> hvs_inverterAirCompressor_wasteHeat_power/1
  Gain2/1 -> Subtract/1, Switch/2, motor mode/2
  Subtract1/1 -> W_to_kW/1
  efficiency/1 -> Product2/1, Subtract1/1
  Constant1/1 -> Switch/3
  Avoid_Div_by_zero/1(1/U) -> Product1/2, Product2/2
  Switch/1 -> efficiency/1, Subtract1/2  "phys_current_A"
  Gain1/1 -> hvs_InverterAirCompressor_hvVoltage/1
  hvsaux_EmotAirCompressor_Voltage_Rq/1 -> motor mode/3
  Saturation/1 -> hvs_emot_AirCompressor_angVel/1, Gain3/1
  Discrete-Time Integrator/1 -> Saturation/1
  Product3/1 -> Rate Transition/1, hvs_emot_AirCompressor_angAcc/1
  Constant5/1 -> Product3/2  "phys_inertia_kgm2"
  Subtract/1 -> Product3/1
  hvs_emot_AirCompressor_torque/1 -> Subtract/2
  Discrete Filter/1 -> Gain2/1
  motor mode/1 -> Switch/1  "ElecMac_ElecPwr_W"
  hvsAux_InverterAirCompressor_torque_Rq/1 -> Discrete Filter/1
  Constant2/1 -> hvs_emot_AirCompressor_angPos/1
  Rate Transition/1 -> Discrete-Time Integrator/1
  [angVel] -> Rate Transition1/1
  Rate Transition1/1 -> motor mode/1
  Switch1/1 -> hvs_InverterAirCompressor_hvCurrent/1

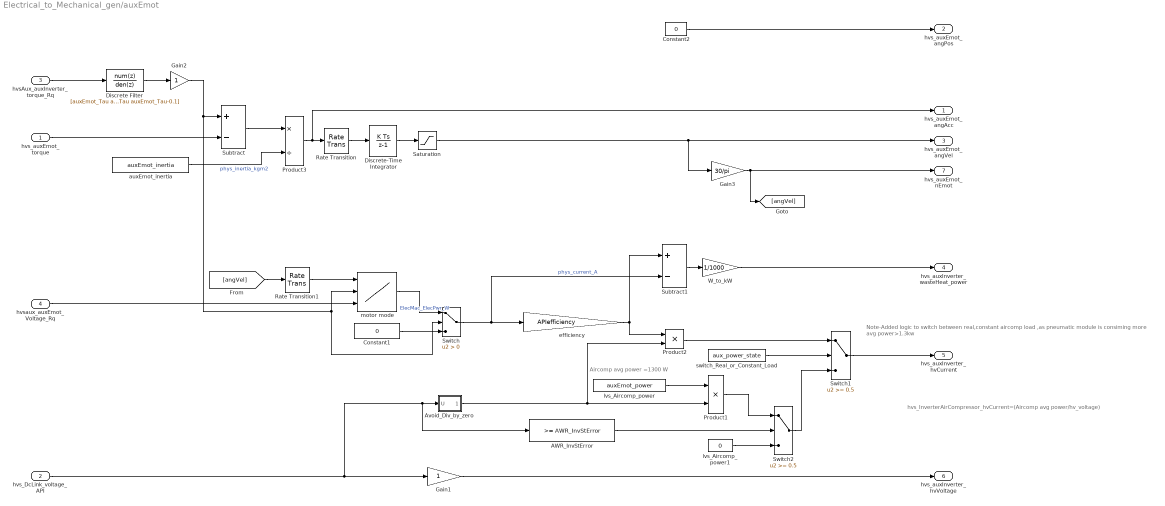
== system Electrical_to_Mechanical_gen/auxEmot ==
  note: Aircomp avg power =1300 W
  note: hvs_InverterAirCompressor_hvCurrent=(Aircomp avg power/hv_voltage)
  note: Note-Added logic to switch between real,constant aircomp load ,as pneumatic module is consiming more avg power>1.3kw
  hvs_auxEmot_torque : Inport
  hvs_DcLink_voltage_API : Inport  Port=2
  hvsAux_auxInverter_torque_Rq : Inport  Port=3
  hvsaux_auxEmot_Voltage_Rq : Inport  Port=4
  AWR_InvStError : simulink/Logic and Bit Operations/Compare To Constant  relop=>=  const=AWR_InvStError  OutDataTypeStr=boolean
  Avoid_Div_by_zero : Subsystem
  Constant1 : Constant  Value=0
  Constant2 : Constant  Value=0
  Discrete Filter : DiscreteFilter  Numerator=[auxEmot_Tau auxEmot_Tau]  Denominator=[0.1+auxEmot_Tau auxEmot_Tau-0.1]
  Discrete-Time Integrator : DiscreteIntegrator  SampleTime=-1  ICPrevOutput=DiscIntNeverNeededParam  ICPrevScaledInput=DiscIntNeverNeededParam
  Gain1 : Gain
      settings: AttributesFormatString=%<Description>
  Gain2 : Gain
      mask init:
      | K = str2num(get_param(bdroot,'FixedStep'));
  Gain3 : Gain  Gain=30/pi
      settings: AttributesFormatString=%<Description>
  Product1 : Product  Inputs=**  RndMeth=Zero
  Product2 : Product  Inputs=**  RndMeth=Zero
  Product3 : Product  Inputs=*/  RndMeth=Zero
  Rate Transition : RateTransition
  Rate Transition1 : RateTransition
  Saturation : Saturate  UpperLimit=inf  LowerLimit=0
  Subtract : Sum  Inputs=+-
  Subtract1 : Sum  Inputs=+-
  Switch : Switch  Criteria=u2 > Threshold
  Switch1 : Switch  Threshold=0.5
  Switch2 : Switch  Threshold=0.5
  W_to_kW : Gain  Gain=1/1000
      settings: AttributesFormatString=%<Description>
  auxEmot_inertia : Constant  Value=auxEmot_inertia
  efficiency : Gain  Gain=APIefficiency
      settings: AttributesFormatString=%<Description>
  lvs_Aircomp_power : Constant  Value=auxEmot_power
  lvs_Aircomp_power1 : Constant  Value=0
  motor mode : Lookup_n-D  NumberOfTableDimensions=3  BreakpointsForDimension1=auxEmot_nTab_3rdD  BreakpointsForDimension2=auxEmot_trqTab_2ndD  BreakpointsForDimension3=auxEmot_vltTab_1stD  Table=auxEmot_pwrAC  ExtrapMethod=Clip  UseLastTableValue=on  InputSameDT=on
  switch_Real_or_Constant_Load : Constant  Value=aux_power_state
  hvs_auxEmot_angAcc : Outport
  hvs_auxEmot_angPos : Outport  Port=2
  hvs_auxEmot_angVel : Outport  Port=3
  hvs_auxInverter_wasteHeat_power : Outport  Port=4
  hvs_auxInverter_hvCurrent : Outport  Port=5
  hvs_auxInverter_hvVoltage : Outport  Port=6
  hvs_auxEmot_nEmot : Outport  Port=7
  wires:
  Switch1/1 -> hvs_auxInverter_hvCurrent/1
  Rate Transition1/1 -> motor mode/1
  [angVel] -> Rate Transition1/1
  Rate Transition/1 -> Discrete-Time Integrator/1
  Constant2/1 -> hvs_auxEmot_angPos/1
  hvsAux_auxInverter_torque_Rq/1 -> Discrete Filter/1
  motor mode/1 -> Switch/1  "ElecMac_ElecPwr_W"
  Discrete Filter/1 -> Gain2/1
  hvs_auxEmot_torque/1 -> Subtract/2
  Subtract/1 -> Product3/1
  auxEmot_inertia/1 -> Product3/2  "phys_inertia_kgm2"
  Product3/1 -> hvs_auxEmot_angAcc/1, Rate Transition/1
  Discrete-Time Integrator/1 -> Saturation/1
  Saturation/1 -> Gain3/1, hvs_auxEmot_angVel/1
  hvsaux_auxEmot_Voltage_Rq/1 -> motor mode/3
  Gain1/1 -> hvs_auxInverter_hvVoltage/1
  Switch/1 -> efficiency/1, Subtract1/2  "phys_current_A"
  Avoid_Div_by_zero/1(1/U) -> Product2/2, Product1/2
  Constant1/1 -> Switch/3
  efficiency/1 -> Subtract1/1, Product2/1
  Subtract1/1 -> W_to_kW/1
  Gain2/1 -> motor mode/2, Switch/2, Subtract/1
  W_to_kW/1 -> hvs_auxInverter_wasteHeat_power/1
  Gain3/1 -> [angVel], hvs_auxEmot_nEmot/1
  Product2/1 -> Switch1/1
  switch_Real_or_Constant_Load/1 -> Switch1/2
  hvs_DcLink_voltage_API/1 -> AWR_InvStError/1, Avoid_Div_by_zero/1(U), Gain1/1
  lvs_Aircomp_power1/1 -> Switch2/3
  lvs_Aircomp_power/1 -> Product1/1
  AWR_InvStError/1 -> Switch2/2
  Product1/1 -> Switch2/1
  Switch2/1 -> Switch1/3

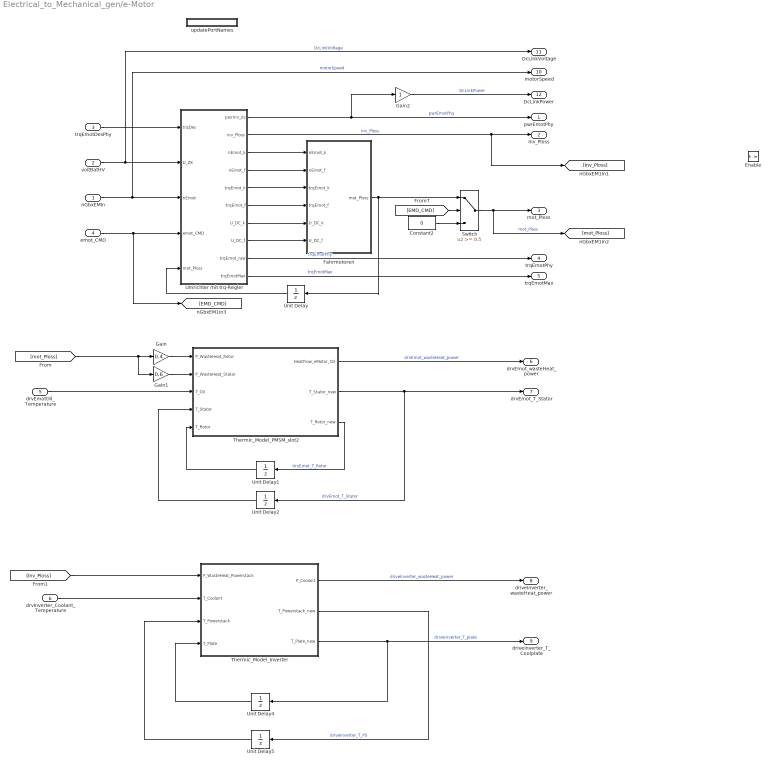
== system Electrical_to_Mechanical_gen/e-Motor ==
  nGbxEMIn : Inport
  voltBatHV : Inport  Port=2
  trqEmotDesPhy : Inport  Port=3
  emot_CMD : Inport  Port=4
  drvEmotOil_Temperature : Inport  Port=5
  drvInverter_Coolant_Temperature : Inport  Port=6
  Enable : EnablePort
  Constant2 : Constant  Value=0
  Fahrmotoren : Subsystem
  Gain : Gain  Gain=0.4
  Gain1 : Gain  Gain=0.6
  Gain2 : Gain
  Switch : Switch  Threshold=0.5
  Thermic_Model_Inverter : Subsystem
  Thermic_Model_PMSM_slot2 : Subsystem
  Umrichter mit trq-Regler : Subsystem
  Unit Delay : UnitDelay  SampleTime=-1
  Unit Delay1 : UnitDelay  InitialCondition=drvEmot_emot_Tstator_init  SampleTime=-1
  Unit Delay2 : UnitDelay  InitialCondition=drvEmot_emot_Trotor_init  SampleTime=-1
  Unit Delay4 : UnitDelay  InitialCondition=drvEmot_inv_Tpowerstack_init  SampleTime=-1
  Unit Delay5 : UnitDelay  InitialCondition=drvEmot_inv_Tplate_init  SampleTime=-1
  updatePortNames : Subsystem
      settings: OpenFcn=std_PortNameFromSignal('Depth',2);
      mask Display: disp('updatePortNames')
  pwrEmotPhy : Outport
  Inv_Ploss : Outport  Port=2
  mot_Ploss : Outport  Port=3
  trqEmotPhy : Outport  Port=4
  trqEmotMax : Outport  Port=5
  drvEmot_wasteHeat_power : Outport  Port=6
  drvEmot_T_Stator : Outport  Port=7
  driveInverter_wasteHeat_power : Outport  Port=8
  driveInverter_T_Coolplate : Outport  Port=9
  motorSpeed : Outport  Port=10
  DcLinkVoltage : Outport  Port=11
  DcLinkPower : Outport  Port=12
  wires:
  Thermic_Model_PMSM_slot2/3(T_Rotor_new) -> Unit Delay1/1  "drvEmot_T_Rotor"
  Unit Delay1/1 -> Thermic_Model_PMSM_slot2/5(T_Rotor)
  Thermic_Model_PMSM_slot2/2(T_Stator_new) -> drvEmot_T_Stator/1, Unit Delay2/1  "drvEmot_T_Stator"
  Unit Delay2/1 -> Thermic_Model_PMSM_slot2/4(T_Stator)
  Gain/1 -> Thermic_Model_PMSM_slot2/1(P_WasteHeat_Rotor)
  Gain1/1 -> Thermic_Model_PMSM_slot2/2(P_WasteHeat_Stator)
  [mot_Ploss] -> Gain1/1, Gain/1
  drvEmotOil_Temperature/1 -> Thermic_Model_PMSM_slot2/3(T_Oil)
  Thermic_Model_PMSM_slot2/1(HeatFlow_eMotor_Oil) -> drvEmot_wasteHeat_power/1  "drvEmot_wasteHeat_power"
  [Inv_Ploss] -> Thermic_Model_Inverter/1(P_WasteHeat_Powerstack)
  Thermic_Model_Inverter/3(T_Plate_new) -> driveInverter_T_Coolplate/1, Unit Delay4/1  "driveInverter_T_plate"
  Unit Delay4/1 -> Thermic_Model_Inverter/4(T_Plate)
  Thermic_Model_Inverter/2(T_Powerstack_new) -> Unit Delay5/1  "driveInverter_T_PS"
  Unit Delay5/1 -> Thermic_Model_Inverter/3(T_Powerstack)
  Thermic_Model_Inverter/1(P_Coolant) -> driveInverter_wasteHeat_power/1  "driveInverter_wasteHeat_power"
  drvInverter_Coolant_Temperature/1 -> Thermic_Model_Inverter/2(T_Coolant)
  Unit Delay/1 -> Umrichter mit trq-Regler/5(mot_Ploss)
  Constant2/1 -> Switch/3
  [EMD_CMD] -> Switch/2
  Fahrmotoren/1(mot_Ploss) -> Switch/1, Unit Delay/1
  emot_CMD/1 -> Umrichter mit trq-Regler/4(emot_CMD), [EMD_CMD]
  Umrichter mit trq-Regler/10(trqEmotMax) -> trqEmotMax/1  "trqEmotMax"
  Umrichter mit trq-Regler/1(pwrInv_dc) -> Gain2/1, pwrEmotPhy/1  "pwrEmotPhy"
  Umrichter mit trq-Regler/2(inv_Ploss) -> [Inv_Ploss], Inv_Ploss/1  "Inv_Ploss"
  Umrichter mit trq-Regler/4(nEmot_f) -> Fahrmotoren/2(nEmot_f)
  Umrichter mit trq-Regler/3(nEmot_k) -> Fahrmotoren/1(nEmot_k)
  Umrichter mit trq-Regler/9(trqEmot_raw) -> trqEmotPhy/1  "trqEmotPhy"
  Umrichter mit trq-Regler/5(trqEmot_k) -> Fahrmotoren/3(trqEmot_k)
  Umrichter mit trq-Regler/6(trqEmot_f) -> Fahrmotoren/4(trqEmot_f)
  Umrichter mit trq-Regler/7(U_DC_k) -> Fahrmotoren/5(U_DC_k)
  Umrichter mit trq-Regler/8(U_DC_f) -> Fahrmotoren/6(U_DC_f)
  Switch/1 -> mot_Ploss/1, [mot_Ploss]  "mot_Ploss"
  nGbxEMIn/1 -> motorSpeed/1, Umrichter mit trq-Regler/3(nEmot)  "motorSpeed"
  voltBatHV/1 -> DcLinkVoltage/1, Umrichter mit trq-Regler/2(U_ZK)  "DcLinkVoltage"
  trqEmotDesPhy/1 -> Umrichter mit trq-Regler/1(trqDes)
  Gain2/1 -> DcLinkPower/1  "DcLinkPower"

== system Electrical_to_Mechanical_gen/EDB_DriveEmot/EMD1_Selection ==
  pti_EMD1_TrqReq_Nm : Inport
  pti_EMD1_ControlMode : Inport  Port=2
  edcu_EMD1_CMD_TorqueRefLim : Inport  Port=3
  edcu_EMD1_CMD_ControlMode : Inport  Port=4
  Bus Creator1 : BusCreator  Inputs=2
  Bus Creator2 : BusCreator  Inputs=2
  Constant2 : Constant  Value=0
  Constant3 : Constant  Value=-1
  Constant4 : Constant  Value=drvEmot_RefTqeMOT
  Logical Operator : Logic  Operator=NOT  AllPortsSameDT=off  OutDataTypeStr=boolean
  Logical Operator1 : Logic  AllPortsSameDT=off  OutDataTypeStr=boolean
  Relational Operator2 : RelationalOperator  Operator===  OutDataTypeStr=boolean
  Relational Operator3 : RelationalOperator  Operator===  OutDataTypeStr=boolean
  Switch : Switch  Criteria=u2 > Threshold
  percent_to_Nm2 : Subsystem
  Signal : Outport
  wires:
  Logical Operator/1 -> Switch/2
  Bus Creator1/1 -> Switch/1
  Logical Operator1/1 -> Logical Operator/1
  percent_to_Nm2/1(Torque_Nm) -> Bus Creator2/1  "EMD1_TrqReq_Nm"
  Constant4/1 -> percent_to_Nm2/2(Reference_Torque)
  pti_EMD1_TrqReq_Nm/1 -> Bus Creator1/1, Relational Operator2/1  "EMD1_TrqReq_Nm"
  pti_EMD1_ControlMode/1 -> Relational Operator3/2, Bus Creator1/2  "EMD1_ControlMode"
  Bus Creator2/1 -> Switch/3
  edcu_EMD1_CMD_TorqueRefLim/1 -> percent_to_Nm2/1(Percentage_Torque)
  Switch/1 -> Signal/1
  edcu_EMD1_CMD_ControlMode/1 -> Bus Creator2/2  "EMD1_ControlMode"
  Relational Operator3/1 -> Logical Operator1/2
  Constant3/1 -> Relational Operator3/1
  Relational Operator2/1 -> Logical Operator1/1
  Constant2/1 -> Relational Operator2/2

== system Electrical_to_Mechanical_gen/EDB_DriveEmot/EMD2_Selection ==
  pti_EMD2_TrqReq_Nm : Inport
  pti_EMD2_ControlMode : Inport  Port=2
  edcu_EMD2_CMD_TorqueRefLim : Inport  Port=3
  edcu_EMD2_CMD_ControlMode : Inport  Port=4
  Bus Creator1 : BusCreator  Inputs=2
  Bus Creator2 : BusCreator  Inputs=2
  Constant2 : Constant  Value=0
  Constant3 : Constant  Value=-1
  Constant4 : Constant  Value=drvEmot_RefTqeMOT
  Logical Operator : Logic  Operator=NOT  AllPortsSameDT=off  OutDataTypeStr=boolean
  Logical Operator1 : Logic  AllPortsSameDT=off  OutDataTypeStr=boolean
  Relational Operator2 : RelationalOperator  Operator===  OutDataTypeStr=boolean
  Relational Operator3 : RelationalOperator  Operator===  OutDataTypeStr=boolean
  Switch : Switch  Criteria=u2 > Threshold
  percent_to_Nm2 : Subsystem
  Signal : Outport
  wires:
  Logical Operator/1 -> Switch/2
  Bus Creator1/1 -> Switch/1
  Logical Operator1/1 -> Logical Operator/1
  percent_to_Nm2/1(Torque_Nm) -> Bus Creator2/1  "EMD2_TrqReq_Nm"
  Constant4/1 -> percent_to_Nm2/2(Reference_Torque)
  pti_EMD2_TrqReq_Nm/1 -> Bus Creator1/1, Relational Operator2/1  "EMD2_TrqReq_Nm"
  pti_EMD2_ControlMode/1 -> Relational Operator3/2, Bus Creator1/2  "EMD2_ControlMode"
  Bus Creator2/1 -> Switch/3
  edcu_EMD2_CMD_TorqueRefLim/1 -> percent_to_Nm2/1(Percentage_Torque)
  Switch/1 -> Signal/1
  edcu_EMD2_CMD_ControlMode/1 -> Bus Creator2/2  "EMD2_ControlMode"
  Relational Operator3/1 -> Logical Operator1/2
  Constant3/1 -> Relational Operator3/1
  Relational Operator2/1 -> Logical Operator1/1
  Constant2/1 -> Relational Operator2/2

== system Electrical_to_Mechanical_gen/EDB_DriveEmot/EMD3_Selection ==
  pti_EMD2_TrqReq_Nm : Inport
  pti_EMD2_ControlMode : Inport  Port=2
  edcu_EMD2_CMD_TorqueRefLim : Inport  Port=3
  edcu_EMD2_CMD_ControlMode : Inport  Port=4
  Bus Creator1 : BusCreator  Inputs=2
  Bus Creator2 : BusCreator  Inputs=2
  Constant2 : Constant  Value=0
  Constant3 : Constant  Value=-1
  Constant4 : Constant  Value=drvEmot_RefTqeMOT
  Logical Operator : Logic  Operator=NOT  AllPortsSameDT=off  OutDataTypeStr=boolean
  Logical Operator1 : Logic  AllPortsSameDT=off  OutDataTypeStr=boolean
  Relational Operator2 : RelationalOperator  Operator===  OutDataTypeStr=boolean
  Relational Operator3 : RelationalOperator  Operator===  OutDataTypeStr=boolean
  Switch : Switch  Criteria=u2 > Threshold
  percent_to_Nm2 : Subsystem
  Signal : Outport
  wires:
  Logical Operator/1 -> Switch/2
  Constant2/1 -> Relational Operator2/2
  Relational Operator2/1 -> Logical Operator1/1
  Constant3/1 -> Relational Operator3/1
  Relational Operator3/1 -> Logical Operator1/2
  edcu_EMD2_CMD_ControlMode/1 -> Bus Creator2/2  "EMD2_ControlMode"
  Switch/1 -> Signal/1
  edcu_EMD2_CMD_TorqueRefLim/1 -> percent_to_Nm2/1(Percentage_Torque)
  Bus Creator2/1 -> Switch/3
  pti_EMD2_ControlMode/1 -> Bus Creator1/2, Relational Operator3/2  "EMD2_ControlMode"
  pti_EMD2_TrqReq_Nm/1 -> Relational Operator2/1, Bus Creator1/1  "EMD2_TrqReq_Nm"
  Constant4/1 -> percent_to_Nm2/2(Reference_Torque)
  percent_to_Nm2/1(Torque_Nm) -> Bus Creator2/1  "EMD2_TrqReq_Nm"
  Logical Operator1/1 -> Logical Operator/1
  Bus Creator1/1 -> Switch/1

== system Electrical_to_Mechanical_gen/EDB_DriveEmot/EMD4_Selection ==
  pti_EMD4_TrqReq_Nm : Inport
  pti_EMD4_ControlMode : Inport  Port=2
  edcu_EMD4_CMD_TorqueRefLim : Inport  Port=3
  edcu_EMD4_CMD_ControlMode : Inport  Port=4
  Bus Creator1 : BusCreator  Inputs=2
  Bus Creator2 : BusCreator  Inputs=2
  Constant2 : Constant  Value=0
  Constant3 : Constant  Value=-1
  Constant4 : Constant  Value=drvEmot_RefTqeMOT
  Logical Operator : Logic  Operator=NOT  AllPortsSameDT=off  OutDataTypeStr=boolean
  Logical Operator1 : Logic  AllPortsSameDT=off  OutDataTypeStr=boolean
  Relational Operator2 : RelationalOperator  Operator===  OutDataTypeStr=boolean
  Relational Operator3 : RelationalOperator  Operator===  OutDataTypeStr=boolean
  Switch : Switch  Criteria=u2 > Threshold
  percent_to_Nm2 : Subsystem
  Signal : Outport
  wires:
  Logical Operator/1 -> Switch/2
  Constant2/1 -> Relational Operator2/2
  Relational Operator2/1 -> Logical Operator1/1
  Constant3/1 -> Relational Operator3/1
  Relational Operator3/1 -> Logical Operator1/2
  edcu_EMD4_CMD_ControlMode/1 -> Bus Creator2/2  "EMD4_ControlMode"
  Switch/1 -> Signal/1
  edcu_EMD4_CMD_TorqueRefLim/1 -> percent_to_Nm2/1(Percentage_Torque)
  Bus Creator2/1 -> Switch/3
  pti_EMD4_ControlMode/1 -> Bus Creator1/2, Relational Operator3/2  "EMD4_ControlMode"
  pti_EMD4_TrqReq_Nm/1 -> Relational Operator2/1, Bus Creator1/1  "EMD4_TrqReq_Nm"
  Constant4/1 -> percent_to_Nm2/2(Reference_Torque)
  percent_to_Nm2/1(Torque_Nm) -> Bus Creator2/1  "EMD4_TrqReq_Nm"
  Logical Operator1/1 -> Logical Operator/1
  Bus Creator1/1 -> Switch/1

== system Electrical_to_Mechanical_gen/EDB_DriveEmot/Emot1_4 ==
  hvs_emot_Emot1_angVel : Inport
  voltBatHV1 : Inport  Port=2
  trqEmotDesPhy1 : Inport  Port=3
  emot_CMD1 : Inport  Port=4
  voltBatHV4 : Inport  Port=5
  trqEmotDesPhy4 : Inport  Port=6
  emot_CMD4 : Inport  Port=7
  hvs_drvEmot1Oil_Temperature : Inport  Port=8
  inv_coolant_temperature : Inport  Port=9
  Emot1_Selection : Inport  Port=10
  Emot4_Selection : Inport  Port=11
  hvs_emot_Emot4_angVel : Inport  Port=12
  hvs_drvEmot4Oil_Temperature : Inport  Port=13
  Bus Creator1 : BusCreator  Inputs=12
  Bus Creator2 : BusCreator  Inputs=12
  Bus Creator3 : BusCreator  Inputs=2
  e-Motor1 : Electrical_to_Mechanical_gen/e-Motor  SystemSampleTime=-1
  e-Motor4 : Electrical_to_Mechanical_gen/e-Motor  SystemSampleTime=-1
  emot1_4B : Outport
  wires:
  e-Motor4/11 -> Bus Creator2/11
  e-Motor4/12 -> Bus Creator2/12
  e-Motor1/12 -> Bus Creator1/12
  e-Motor1/11 -> Bus Creator1/11
  e-Motor4/10 -> Bus Creator2/10
  e-Motor1/10 -> Bus Creator1/10
  hvs_drvEmot4Oil_Temperature/1 -> e-Motor4/5
  Emot1_Selection/1 -> e-Motor1/Enable
  Emot4_Selection/1 -> e-Motor4/Enable
  Bus Creator3/1 -> emot1_4B/1  "emot1_4B"
  trqEmotDesPhy4/1 -> e-Motor4/3
  Bus Creator2/1 -> Bus Creator3/2  "emot4B"
  Bus Creator1/1 -> Bus Creator3/1  "emot1B"
  voltBatHV4/1 -> e-Motor4/2
  hvs_emot_Emot4_angVel/1 -> e-Motor4/1
  voltBatHV1/1 -> e-Motor1/2
  trqEmotDesPhy1/1 -> e-Motor1/3
  hvs_emot_Emot1_angVel/1 -> e-Motor1/1
  e-Motor1/3 -> Bus Creator1/3
  e-Motor1/4 -> Bus Creator1/4
  e-Motor1/1 -> Bus Creator1/1
  e-Motor1/2 -> Bus Creator1/2
  e-Motor1/5 -> Bus Creator1/5
  e-Motor4/1 -> Bus Creator2/1
  e-Motor4/2 -> Bus Creator2/2
  e-Motor4/3 -> Bus Creator2/3
  e-Motor4/4 -> Bus Creator2/4
  e-Motor4/5 -> Bus Creator2/5
  emot_CMD1/1 -> e-Motor1/4
  emot_CMD4/1 -> e-Motor4/4
  inv_coolant_temperature/1 -> e-Motor4/6, e-Motor1/6
  hvs_drvEmot1Oil_Temperature/1 -> e-Motor1/5
  e-Motor1/6 -> Bus Creator1/6
  e-Motor1/7 -> Bus Creator1/7
  e-Motor1/9 -> Bus Creator1/9
  e-Motor1/8 -> Bus Creator1/8
  e-Motor4/6 -> Bus Creator2/6
  e-Motor4/7 -> Bus Creator2/7
  e-Motor4/8 -> Bus Creator2/8
  e-Motor4/9 -> Bus Creator2/9
